simulink model "LQR_Desired_Command_Accel"  (R2024a)
settings: Solver=FixedStepDiscrete  StartTime=0.0  StopTime=10.0  FixedStep=0.05  RelTol=1e-3
undefined symbols (not defined in the file): simStepSize
settings Model: Creator=darkh  LastModifiedBy=darkh
settings OptimizationCC: ZeroExternalMemoryAtStartup=off  ZeroInternalMemoryAtStartup=off
settings RTWCC: Description=Generate an RTMaps component embedding the model  SystemTargetFile=rtmaps.tlc  TemplateMakefile=rtmaps_default_tmf  PostCodeGenCommand=rtmaps_post_code_generation(buildInfo)  RetainRTWFile=on  TargetLang=C++
settings STFCustomTargetCC: TargetLangStandard=C++11 (ISO)  ModelReferenceCompliant=off  ConcurrentExecutionCompliant=on  CombineOutputUpdateFcns=on  CodeInterfacePackaging=C++ class  CPPClassGenCompliant=on  GRTInterface=off  UseToolchainInfoCompliant=off  SystemTargetFile=rtmaps.tlc
settings GRTTargetCC: TargetLangStandard=C++11 (ISO)  ModelReferenceCompliant=off  ParMdlRefBuildCompliant=off  CompOptLevelCompliant=off  MatFileLogging=off  CodeInterfacePackaging=C++ class  UseToolchainInfoCompliant=off

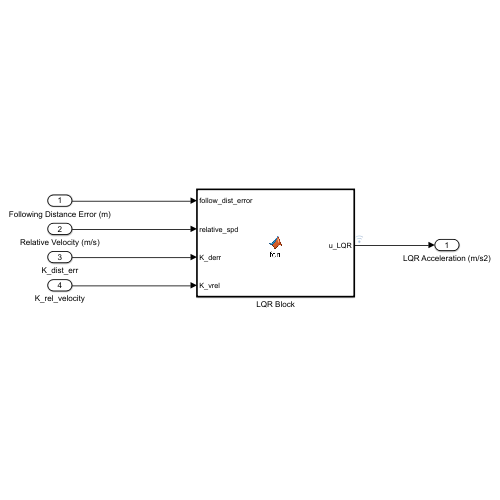
[thumbnail: Simulink's stored preview of the top-level diagram]
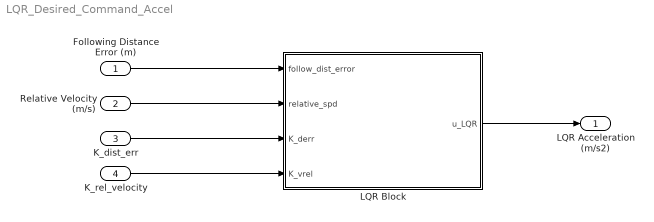
== system LQR_Desired_Command_Accel ==
  Following Distance Error (m) : Inport
  Relative Velocity (m/s) : Inport  Port=2
  K_dist_err : Inport  Port=3
  K_rel_velocity : Inport  Port=4
  LQR Block : MATLAB Function  TreatAsAtomicUnit=on  SystemSampleTime=simStepSize
  LQR Acceleration (m/s2) : Outport
  wires:
  LQR Block/1(u_LQR) -> LQR Acceleration (m/s2)/1
  Following Distance Error (m)/1 -> LQR Block/1(follow_dist_error)
  Relative Velocity (m/s)/1 -> LQR Block/2(relative_spd)
  K_dist_err/1 -> LQR Block/3(K_derr)
  K_rel_velocity/1 -> LQR Block/4(K_vrel)

== matlab function LQR_Desired_Command_Accel/LQR Block ==
  data: follow_dist_error input; relative_spd input; u_LQR output; K_derr input; K_vrel input
 function u_LQR = fcn(follow_dist_error, relative_spd, K_derr, K_vrel)
u_LQR = -K_derr*follow_dist_error-K_vrel*relative_spd;
